simulink model "UAV_rate_dynamics"  (R2016a)
settings: Solver=VariableStepAuto  StartTime=0.0  StopTime=10.0  RelTol=1e-3
values from neighbouring files (symbols this model uses):
  I = 1e-6 .* [16.6 0.83 0.72 ... (first row only)    [init_UAV_model.m]
  omega0 = [0;0;0]    [init_UAV_model.m]
settings Model: Creator=mgreiff  LastModifiedBy=mgreiff

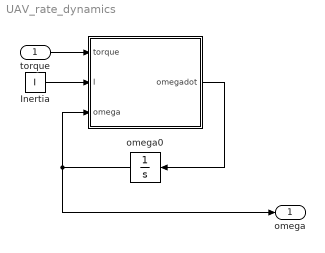
== system UAV_rate_dynamics ==
  torque : Inport  PortDimensions=3
  " " : MATLAB Function  TreatAsAtomicUnit=on
  Inertia : Constant  Value=I
  omega0 : Integrator  InitialCondition=omega0
  omega : Outport  PortDimensions=3
  wires:
  " "/1(omegadot) -> omega0/1
  omega0/1 -> omega/1, " "/3(omega)
  Inertia/1 -> " "/2(I)
  torque/1 -> " "/1(torque)

== matlab function UAV_rate_dynamics/  ==
  data: torque input; I input; omegadot output; omega input
function omegadot  = f(torque, I, omega)
% ~~~ Copyright (c) 2018 Marcus Greiff (see LICENCE.md) ~~~
%
% Model of the attitude rate dynamics, a subset of the UAV dynamics
%
%    omegadot  = f(torque, I, omega)
%
% The inputs to this subsystem are the torques, and the equations are
% parametrized by an inertial tensor I which i assumed to be positive
% definite and symmetric. Omega denotes the attitude rate defined in the
% body frame of reference.
omegadot = I\(torque - skew(omega)*(I*omega));
end

function S = skew(v)
    vx = v(1);
    vy = v(2);
    vz = v(3);
    S = [0 -vz vy; vz 0 -vx; -vy vx 0];
end
